simulink model "difflinrelay"  (Simulink 8.5)
settings: Solver=ode45  StartTime=0.0  StopTime=0.01  RelTol=1e-3
values from neighbouring files (symbols this model uses):
  n = abs(fix(dif/360))    [DE_12.m]
undefined symbols (not defined in the file or in its folder): b, den, dx, flagc, m, minx, num
libraries: elements x21, simulink_extras x9
(part 1 of 2)
settings Model: Creator=PC  LastModifiedBy=PC  ExtModeTrigMode=oneshot  ExtModeArmWhenConnect=off
settings DataIOCC: LimitDataPoints=off
settings OptimizationCC: BlockReduction=off  BooleanDataType=off  ExpressionDepthLimit=128
settings DebuggingCC: SaveWithParameterizedLinksMsg=none  SignalResolutionControl=TryResolveAllWithWarning  MultiTaskDSMMsg=warning  MultiTaskCondExecSysMsg=none  FcnCallInpInsideContextMsg=EnableAllAsError  StateNameClashWarn=none  StrictBusMsg=None
settings HardwareCC: TargetUnknown=on

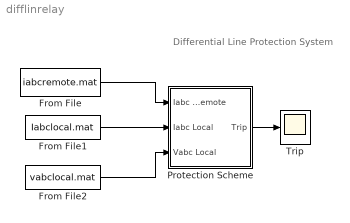
== system difflinrelay ==
  note: Differential Line Protection System
  From File : FromFile  FileName=iabcremote.mat  SampleTime=0
  From File1 : FromFile  FileName=Iabclocal.mat  SampleTime=0
  From File2 : FromFile  FileName=vabclocal.mat  SampleTime=0
  Protection Scheme : Subsystem  mask{bias=[ 0 0;1 0.5 ;3 0.8; 5 4; 7 4.2 ; 8 4.22], Cpg=1e-6, Cpp=1e-7, zone1=[0 0 ;1 0; 1 1; 0.5 1], zone2=[0 0; 2 0; 2 2; 0 2], zone3=[0 0; 3 0; 3 3 ;0 3], zone4=[0 0; 4 0; 5 4; 1 5], reversezone=[0 0; -1 0; -1 -1; 0 -1], delay=[0.001 0.002 0.003 0.001]}
      mask prompts: bias "Bias Characteristic"; Cpg "Capacitance between phase and ground (F)"; Cpp "Mutual Capacitance between phases (F)"; zone1 "Back-up protection zone 1:"; zone2 "Back-up protection zone 2"; zone3 "Back-up protection zone 3"; zone4 "Back-up protection zone 4"; reversezone "Back-up protection reverse zone"; delay "Delay times for zone protection [Z2 Z3 Z4 Reverse]"
  Trip : Scope
      settings: TickLabels=on  TimeRange=0.01  YMin=0  YMax=1.5
  wires:
  Protection Scheme/1(Trip) -> Trip/1
  From File2/1 -> Protection Scheme/3(Vabc Local)
  From File1/1 -> Protection Scheme/2(Iabc Local)
  From File/1 -> Protection Scheme/1(Iabc Remote)

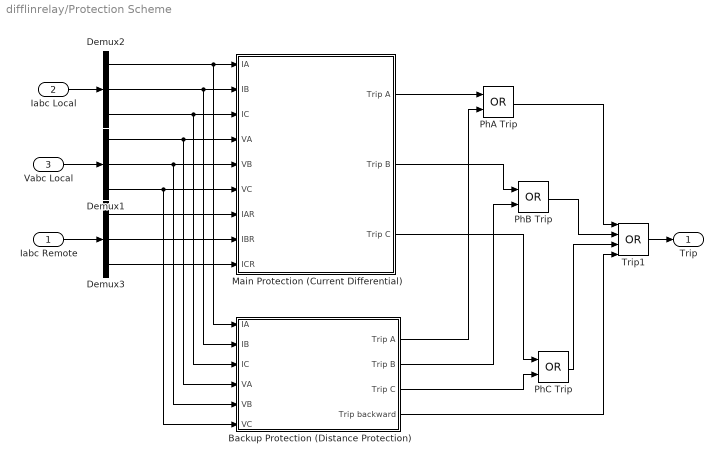
== system difflinrelay/Protection Scheme ==
  Iabc Remote : Inport
  Iabc Local : Inport  Port=2
  Vabc Local : Inport  Port=3
  Backup Protection (Distance Protection) : Subsystem
  Demux1 : Demux  Outputs=3
  Demux2 : Demux  Outputs=3
  Demux3 : Demux  Outputs=3
  Main Protection (Current Differential) : Subsystem
  PhA Trip : Logic  Operator=OR
  PhB Trip : Logic  Operator=OR
  PhC Trip : Logic  Operator=OR
  Trip1 : Logic  Operator=OR  Inputs=4
  Trip : Outport
  wires:
  Vabc Local/1 -> Demux1/1
  Iabc Local/1 -> Demux2/1
  Iabc Remote/1 -> Demux3/1
  Trip1/1 -> Trip/1
  PhA Trip/1 -> Trip1/1
  PhB Trip/1 -> Trip1/2
  PhC Trip/1 -> Trip1/3
  Backup Protection (Distance Protection)/1(Trip A) -> PhA Trip/2
  Backup Protection (Distance Protection)/2(Trip B) -> PhB Trip/2
  Backup Protection (Distance Protection)/3(Trip C) -> PhC Trip/2
  Main Protection (Current Differential)/1(Trip A) -> PhA Trip/1
  Main Protection (Current Differential)/2(Trip B) -> PhB Trip/1
  Main Protection (Current Differential)/3(Trip C) -> PhC Trip/1
  Demux3/1 -> Main Protection (Current Differential)/7(IAR)
  Demux3/2 -> Main Protection (Current Differential)/8(IBR)
  Demux3/3 -> Main Protection (Current Differential)/9(ICR)
  Demux2/1 -> Main Protection (Current Differential)/1(IA), Backup Protection (Distance Protection)/1(IA)
  Demux2/2 -> Main Protection (Current Differential)/2(IB), Backup Protection (Distance Protection)/2(IB)
  Demux2/3 -> Main Protection (Current Differential)/3(IC), Backup Protection (Distance Protection)/3(IC)
  Demux1/1 -> Main Protection (Current Differential)/4(VA), Backup Protection (Distance Protection)/4(VA)
  Demux1/2 -> Main Protection (Current Differential)/5(VB), Backup Protection (Distance Protection)/5(VB)
  Demux1/3 -> Main Protection (Current Differential)/6(VC), Backup Protection (Distance Protection)/6(VC)
  Backup Protection (Distance Protection)/4(Trip backward) -> Trip1/4

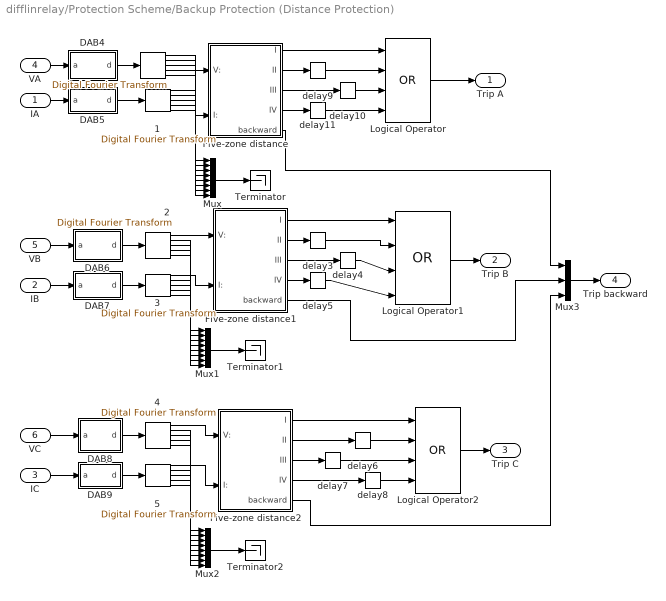
== system difflinrelay/Protection Scheme/Backup Protection (Distance Protection) ==
  IA : Inport
  IB : Inport  Port=2
  IC : Inport  Port=3
  VA : Inport  Port=4
  VB : Inport  Port=5
  VC : Inport  Port=6
   {,1..5} (6 alike) : elements/   fo=60  window_size=40  harmonic=[1 2 3 4 5]
  DAB4 : Subsystem  mask(Data Adquisition Board){filter=off, approx=Bessel, order=2, numerator=[], denominator=[], freq=180, resdis=off, vertres=12, xmax=10, winsize=40, G=1.0, fs=60*40}
      mask prompts: filter "Disable Analog Filter"; approx "Filter approximation"; numerator "Free expression filter: numerator(descending order of s)"; denominator "Free expression filter: denominator:"; freq "Cut-off frequency"; resdis "Disable Vertical Resolution"; vertres "Vertical Resolution: No. of bits"; xmax "Vertical Resolution: signal range"; winsize "Window size"; G "Gain"; fs "Sampling frequency"
      mask help: Performs analog filtering, signal conditioning and sampling. A single signal is the input, a buffer with the signal samples is the output. The options include analog filter enable/disable switch, type, order and cut-off frequency of the analog filter, conditioning gain, sampling frequency, number of bits, the length of the buffer.
      mask init:
      | dab1
      mask TypeOptions approx: Bessel | Tschebyscheff | Butterworth | free expression
      mask TypeOptions order: 2 | 3 | 4
      mask TypeOptions vertres: 8 | 12 | 16
      mask Display: disp('DAB')
  DAB5 : Subsystem  mask(Data Adquisition Board){filter=off, approx=Bessel, order=2, numerator=[], denominator=[], freq=180, resdis=off, vertres=12, xmax=10, winsize=40, G=1.0, fs=60*40}
      mask prompts: filter "Disable Analog Filter"; approx "Filter approximation"; numerator "Free expression filter: numerator(descending order of s)"; denominator "Free expression filter: denominator:"; freq "Cut-off frequency"; resdis "Disable Vertical Resolution"; vertres "Vertical Resolution: No. of bits"; xmax "Vertical Resolution: signal range"; winsize "Window size"; G "Gain"; fs "Sampling frequency"
      mask help: Performs analog filtering, signal conditioning and sampling. A single signal is the input, a buffer with the signal samples is the output. The options include analog filter enable/disable switch, type, order and cut-off frequency of the analog filter, conditioning gain, sampling frequency, number of bits, the length of the buffer.
      mask init:
      | dab1
      mask TypeOptions approx: Bessel | Tschebyscheff | Butterworth | free expression
      mask TypeOptions order: 2 | 3 | 4
      mask TypeOptions vertres: 8 | 12 | 16
      mask Display: disp('DAB')
  DAB6 : Subsystem  mask(Data Adquisition Board){filter=off, approx=Bessel, order=2, numerator=[], denominator=[], freq=180, resdis=off, vertres=12, xmax=10, winsize=40, G=1.0, fs=60*40}
      mask prompts: filter "Disable Analog Filter"; approx "Filter approximation"; numerator "Free expression filter: numerator(descending order of s)"; denominator "Free expression filter: denominator:"; freq "Cut-off frequency"; resdis "Disable Vertical Resolution"; vertres "Vertical Resolution: No. of bits"; xmax "Vertical Resolution: signal range"; winsize "Window size"; G "Gain"; fs "Sampling frequency"
      mask help: Performs analog filtering, signal conditioning and sampling. A single signal is the input, a buffer with the signal samples is the output. The options include analog filter enable/disable switch, type, order and cut-off frequency of the analog filter, conditioning gain, sampling frequency, number of bits, the length of the buffer.
      mask init:
      | dab1
      mask TypeOptions approx: Bessel | Tschebyscheff | Butterworth | free expression
      mask TypeOptions order: 2 | 3 | 4
      mask TypeOptions vertres: 8 | 12 | 16
      mask Display: disp('DAB')
  DAB7 : Subsystem  mask(Data Adquisition Board){filter=off, approx=Bessel, order=2, numerator=[], denominator=[], freq=180, resdis=off, vertres=12, xmax=10, winsize=40, G=1.0, fs=60*40}
      mask prompts: filter "Disable Analog Filter"; approx "Filter approximation"; numerator "Free expression filter: numerator(descending order of s)"; denominator "Free expression filter: denominator:"; freq "Cut-off frequency"; resdis "Disable Vertical Resolution"; vertres "Vertical Resolution: No. of bits"; xmax "Vertical Resolution: signal range"; winsize "Window size"; G "Gain"; fs "Sampling frequency"
      mask help: Performs analog filtering, signal conditioning and sampling. A single signal is the input, a buffer with the signal samples is the output. The options include analog filter enable/disable switch, type, order and cut-off frequency of the analog filter, conditioning gain, sampling frequency, number of bits, the length of the buffer.
      mask init:
      | dab1
      mask TypeOptions approx: Bessel | Tschebyscheff | Butterworth | free expression
      mask TypeOptions order: 2 | 3 | 4
      mask TypeOptions vertres: 8 | 12 | 16
      mask Display: disp('DAB')
  DAB8 : Subsystem  mask(Data Adquisition Board){filter=off, approx=Bessel, order=2, numerator=[], denominator=[], freq=180, resdis=off, vertres=12, xmax=10, winsize=40, G=1.0, fs=60*40}
      mask prompts: filter "Disable Analog Filter"; approx "Filter approximation"; numerator "Free expression filter: numerator(descending order of s)"; denominator "Free expression filter: denominator:"; freq "Cut-off frequency"; resdis "Disable Vertical Resolution"; vertres "Vertical Resolution: No. of bits"; xmax "Vertical Resolution: signal range"; winsize "Window size"; G "Gain"; fs "Sampling frequency"
      mask help: Performs analog filtering, signal conditioning and sampling. A single signal is the input, a buffer with the signal samples is the output. The options include analog filter enable/disable switch, type, order and cut-off frequency of the analog filter, conditioning gain, sampling frequency, number of bits, the length of the buffer.
      mask init:
      | dab1
      mask TypeOptions approx: Bessel | Tschebyscheff | Butterworth | free expression
      mask TypeOptions order: 2 | 3 | 4
      mask TypeOptions vertres: 8 | 12 | 16
      mask Display: disp('DAB')
  DAB9 : Subsystem  mask(Data Adquisition Board){filter=off, approx=Bessel, order=2, numerator=[], denominator=[], freq=180, resdis=off, vertres=12, xmax=10, winsize=40, G=1.0, fs=60*40}
      mask prompts: filter "Disable Analog Filter"; approx "Filter approximation"; numerator "Free expression filter: numerator(descending order of s)"; denominator "Free expression filter: denominator:"; freq "Cut-off frequency"; resdis "Disable Vertical Resolution"; vertres "Vertical Resolution: No. of bits"; xmax "Vertical Resolution: signal range"; winsize "Window size"; G "Gain"; fs "Sampling frequency"
      mask help: Performs analog filtering, signal conditioning and sampling. A single signal is the input, a buffer with the signal samples is the output. The options include analog filter enable/disable switch, type, order and cut-off frequency of the analog filter, conditioning gain, sampling frequency, number of bits, the length of the buffer.
      mask init:
      | dab1
      mask TypeOptions approx: Bessel | Tschebyscheff | Butterworth | free expression
      mask TypeOptions order: 2 | 3 | 4
      mask TypeOptions vertres: 8 | 12 | 16
      mask Display: disp('DAB')
  Five-zone distance : Subsystem
  Five-zone distance1 : Subsystem
  Five-zone distance2 : Subsystem
  Logical Operator : Logic  Operator=OR  Inputs=4
  Logical Operator1 : Logic  Operator=OR  Inputs=4
  Logical Operator2 : Logic  Operator=OR  Inputs=4
  Mux : Mux  Inputs=8
  Mux1 : Mux  Inputs=8
  Mux2 : Mux  Inputs=8
  Mux3 : Mux  Inputs=3
  Terminator : Terminator
  Terminator1 : Terminator
  Terminator2 : Terminator
  delay10 : TransportDelay  DelayTime=delay(2)
  delay11 : TransportDelay  DelayTime=delay(3)
  delay3 : TransportDelay  DelayTime=delay(1)
  delay4 : TransportDelay  DelayTime=delay(2)
  delay5 : TransportDelay  DelayTime=delay(3)
  delay6 : TransportDelay  DelayTime=delay(1)
  delay7 : TransportDelay  DelayTime=delay(2)
  delay8 : TransportDelay  DelayTime=delay(3)
  delay9 : TransportDelay  DelayTime=delay(1)
  Trip A : Outport
  Trip B : Outport  Port=2
  Trip C : Outport  Port=3
  Trip backward : Outport  Port=4
  wires:
  Five-zone distance1/1(I) -> Logical Operator1/1
  " 4"/1 -> Five-zone distance2/1(V:)
  DAB9/1(d) -> " 5"/1
  DAB8/1(d) -> " 4"/1
  VC/1 -> DAB8/1(a)
  IC/1 -> DAB9/1(a)
  Logical Operator2/1 -> Trip C/1
  " 2"/1 -> Five-zone distance1/1(V:)
  DAB7/1(d) -> " 3"/1
  DAB6/1(d) -> " 2"/1
  " 3"/1 -> Five-zone distance1/2(I:)
  Five-zone distance1/2(II) -> delay3/1
  Five-zone distance1/3(III) -> delay4/1
  Five-zone distance1/4(IV) -> delay5/1
  delay3/1 -> Logical Operator1/2
  delay4/1 -> Logical Operator1/3
  delay5/1 -> Logical Operator1/4
  VB/1 -> DAB6/1(a)
  IB/1 -> DAB7/1(a)
  Logical Operator1/1 -> Trip B/1
  " "/1 -> Five-zone distance/1(V:)
  DAB5/1(d) -> " 1"/1
  DAB4/1(d) -> " "/1
  " 1"/1 -> Five-zone distance/2(I:)
  Five-zone distance/1(I) -> Logical Operator/1
  VA/1 -> DAB4/1(a)
  IA/1 -> DAB5/1(a)
  Logical Operator/1 -> Trip A/1
  " "/3 -> Mux/1
  " "/2 -> Mux/2
  " "/4 -> Mux/3
  " "/5 -> Mux/4
  " 1"/2 -> Mux/5
  " 1"/3 -> Mux/6
  " 1"/4 -> Mux/7
  " 1"/5 -> Mux/8
  " 2"/2 -> Mux1/1
  " 2"/3 -> Mux1/2
  " 2"/4 -> Mux1/3
  " 2"/5 -> Mux1/4
  " 3"/2 -> Mux1/5
  " 3"/3 -> Mux1/6
  " 3"/4 -> Mux1/7
  " 3"/5 -> Mux1/8
  " 4"/3 -> Mux2/1
  " 4"/2 -> Mux2/2
  " 4"/4 -> Mux2/3
  " 4"/5 -> Mux2/4
  " 5"/2 -> Mux2/5
  " 5"/3 -> Mux2/6
  " 5"/4 -> Mux2/7
  " 5"/5 -> Mux2/8
  Five-zone distance/5(backward) -> Mux3/1
  Five-zone distance1/5(backward) -> Mux3/2
  " 5"/1 -> Five-zone distance2/2(I:)
  delay6/1 -> Logical Operator2/2
  delay7/1 -> Logical Operator2/3
  delay8/1 -> Logical Operator2/4
  Five-zone distance2/1(I) -> Logical Operator2/1
  Five-zone distance2/2(II) -> delay6/1
  Five-zone distance2/3(III) -> delay7/1
  Five-zone distance2/4(IV) -> delay8/1
  Five-zone distance2/5(backward) -> Mux3/3
  Five-zone distance/2(II) -> delay9/1
  delay9/1 -> Logical Operator/2
  Five-zone distance/3(III) -> delay10/1
  Five-zone distance/4(IV) -> delay11/1
  Mux/1 -> Terminator/1
  Mux1/1 -> Terminator1/1
  Mux2/1 -> Terminator2/1
  delay10/1 -> Logical Operator/3
  delay11/1 -> Logical Operator/4
  Mux3/1 -> Trip backward/1

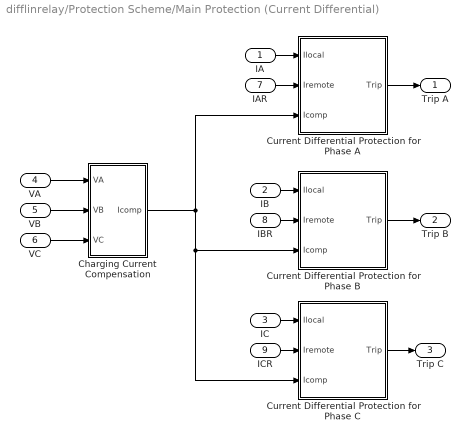
== system difflinrelay/Protection Scheme/Main Protection (Current Differential) ==
  IA : Inport
  IB : Inport  Port=2
  IC : Inport  Port=3
  VA : Inport  Port=4
  VB : Inport  Port=5
  VC : Inport  Port=6
  IAR : Inport  Port=7
  IBR : Inport  Port=8
  ICR : Inport  Port=9
  Charging Current Compensation : Subsystem
  Current Differential Protection for Phase A : Subsystem
  Current Differential Protection for Phase B : Subsystem
  Current Differential Protection for Phase C : Subsystem
  Trip A : Outport  InitialOutput=0
  Trip B : Outport  Port=2  InitialOutput=0
  Trip C : Outport  Port=3  InitialOutput=0
  wires:
  IA/1 -> Current Differential Protection for Phase A/1(Ilocal)
  IAR/1 -> Current Differential Protection for Phase A/2(Iremote)
  IB/1 -> Current Differential Protection for Phase B/1(Ilocal)
  Current Differential Protection for Phase C/1(Trip) -> Trip C/1
  Current Differential Protection for Phase A/1(Trip) -> Trip A/1
  Current Differential Protection for Phase B/1(Trip) -> Trip B/1
  VB/1 -> Charging Current Compensation/2(VB)
  IBR/1 -> Current Differential Protection for Phase B/2(Iremote)
  IC/1 -> Current Differential Protection for Phase C/1(Ilocal)
  VA/1 -> Charging Current Compensation/1(VA)
  VC/1 -> Charging Current Compensation/3(VC)
  ICR/1 -> Current Differential Protection for Phase C/2(Iremote)
  Charging Current Compensation/1(Icomp) -> Current Differential Protection for Phase A/3(Icomp), Current Differential Protection for Phase B/3(Icomp), Current Differential Protection for Phase C/3(Icomp)

== system difflinrelay/Protection Scheme/Backup Protection (Distance Protection)/DAB4 ==
  a : Inport
  AD & Buffer : S-Function  FunctionName=dab2  Parameters=winsize,fs,dx,resdis
  Analog Filter : TransferFcn  Numerator=num  Denominator=den
  Gain : Gain  Gain=G  SaturateOnIntegerOverflow=on  OutDataTypeStr=Inherit: Same as input  ParamDataTypeStr=Inherit: Same as input
  Zero-Order Hold : ZeroOrderHold  SampleTime=1/fs
  d : Outport  InitialOutput=[zeros(winsize,1)]
  wires:
  Analog Filter/1 -> Gain/1
  Gain/1 -> Zero-Order Hold/1
  Zero-Order Hold/1 -> AD & Buffer/1
  a/1 -> Analog Filter/1
  AD & Buffer/1 -> d/1

== system difflinrelay/Protection Scheme/Backup Protection (Distance Protection)/DAB5 ==
  a : Inport
  AD & Buffer : S-Function  FunctionName=dab2  Parameters=winsize,fs,dx,resdis
  Analog Filter : TransferFcn  Numerator=num  Denominator=den
  Gain : Gain  Gain=G  SaturateOnIntegerOverflow=on  OutDataTypeStr=Inherit: Same as input  ParamDataTypeStr=Inherit: Same as input
  Zero-Order Hold : ZeroOrderHold  SampleTime=1/fs
  d : Outport  InitialOutput=[zeros(winsize,1)]
  wires:
  AD & Buffer/1 -> d/1
  a/1 -> Analog Filter/1
  Zero-Order Hold/1 -> AD & Buffer/1
  Gain/1 -> Zero-Order Hold/1
  Analog Filter/1 -> Gain/1

== system difflinrelay/Protection Scheme/Backup Protection (Distance Protection)/DAB6 ==
  a : Inport
  AD & Buffer : S-Function  FunctionName=dab2  Parameters=winsize,fs,dx,resdis
  Analog Filter : TransferFcn  Numerator=num  Denominator=den
  Gain : Gain  Gain=G  SaturateOnIntegerOverflow=on  OutDataTypeStr=Inherit: Same as input  ParamDataTypeStr=Inherit: Same as input
  Zero-Order Hold : ZeroOrderHold  SampleTime=1/fs
  d : Outport  InitialOutput=[zeros(winsize,1)]
  wires:
  AD & Buffer/1 -> d/1
  a/1 -> Analog Filter/1
  Zero-Order Hold/1 -> AD & Buffer/1
  Gain/1 -> Zero-Order Hold/1
  Analog Filter/1 -> Gain/1

== system difflinrelay/Protection Scheme/Backup Protection (Distance Protection)/DAB7 ==
  a : Inport
  AD & Buffer : S-Function  FunctionName=dab2  Parameters=winsize,fs,dx,resdis
  Analog Filter : TransferFcn  Numerator=num  Denominator=den
  Gain : Gain  Gain=G  SaturateOnIntegerOverflow=on  OutDataTypeStr=Inherit: Same as input  ParamDataTypeStr=Inherit: Same as input
  Zero-Order Hold : ZeroOrderHold  SampleTime=1/fs
  d : Outport  InitialOutput=[zeros(winsize,1)]
  wires:
  Analog Filter/1 -> Gain/1
  Gain/1 -> Zero-Order Hold/1
  Zero-Order Hold/1 -> AD & Buffer/1
  a/1 -> Analog Filter/1
  AD & Buffer/1 -> d/1

== system difflinrelay/Protection Scheme/Backup Protection (Distance Protection)/DAB8 ==
  a : Inport
  AD & Buffer : S-Function  FunctionName=dab2  Parameters=winsize,fs,dx,resdis
  Analog Filter : TransferFcn  Numerator=num  Denominator=den
  Gain : Gain  Gain=G  SaturateOnIntegerOverflow=on  OutDataTypeStr=Inherit: Same as input  ParamDataTypeStr=Inherit: Same as input
  Zero-Order Hold : ZeroOrderHold  SampleTime=1/fs
  d : Outport  InitialOutput=[zeros(winsize,1)]
  wires:
  Analog Filter/1 -> Gain/1
  Gain/1 -> Zero-Order Hold/1
  Zero-Order Hold/1 -> AD & Buffer/1
  a/1 -> Analog Filter/1
  AD & Buffer/1 -> d/1

== system difflinrelay/Protection Scheme/Backup Protection (Distance Protection)/DAB9 ==
  a : Inport
  AD & Buffer : S-Function  FunctionName=dab2  Parameters=winsize,fs,dx,resdis
  Analog Filter : TransferFcn  Numerator=num  Denominator=den
  Gain : Gain  Gain=G  SaturateOnIntegerOverflow=on  OutDataTypeStr=Inherit: Same as input  ParamDataTypeStr=Inherit: Same as input
  Zero-Order Hold : ZeroOrderHold  SampleTime=1/fs
  d : Outport  InitialOutput=[zeros(winsize,1)]
  wires:
  AD & Buffer/1 -> d/1
  a/1 -> Analog Filter/1
  Zero-Order Hold/1 -> AD & Buffer/1
  Gain/1 -> Zero-Order Hold/1
  Analog Filter/1 -> Gain/1

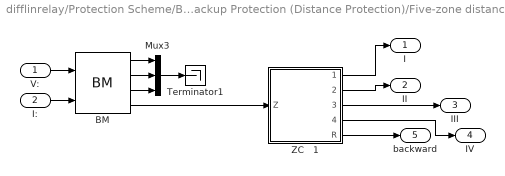
== system difflinrelay/Protection Scheme/Backup Protection (Distance Protection)/Five-zone distance ==
  V: : Inport
  I: : Inport  Port=2
  BM : elements/BM  tpostv=none  plenv=4  tposti=none  pleni=4  tposts=none  plens=4  tpostz=none  plenz=4
  Mux3 : Mux  Inputs=3
  Terminator1 : Terminator
  ZC   1 : Subsystem  mask(Zone Comparator){typez=Free expression, z1=zone1, z2=zone2, z3=zone3, z4=zone4, zr=reversezone, fs=4*60}
      mask prompts: typez "shape"; z1 "Zone 1"; z2 "Zone 2"; z3 "Zone 3"; z4 "Zone 4"; zr "Reverse Zone"; fs "Sampling frecuency (Hz):"
      mask help: This block performs the zone comparison. Its inputs are the resistance and reactance signals. Four forward and one backward zones are implemented. The output that corresponds to the zone where the impedance is located is set to one while the rest of the outputs are zero Either the mho or free expression characteristics may be set. For the mho characteristic, the zones are defined by specifying the center of each circle (all the circles are tangent to the origin). For the free expression, arrays with consecutive vertices specify the polygons for each zone.
      mask init:
      | zc1;
      mask TypeOptions typez: Mho characteristic | Free expression
      mask Display:
      | plot(x1(:,1),x1(:,2));
      | plot(x2(:,1),x2(:,2));
      | plot(x3(:,1),x3(:,2));
      | plot(x4(:,1),x4(:,2));
      | plot(xr(:,1),xr(:,2));
  I : Outport
  II : Outport  Port=2
  III : Outport  Port=3
  IV : Outport  Port=4
  backward : Outport  Port=5
  wires:
  I:/1 -> BM/2
  V:/1 -> BM/1
  BM/4 -> ZC   1/1(Z)
  BM/1 -> Mux3/1
  BM/2 -> Mux3/2
  BM/3 -> Mux3/3
  ZC   1/1(1) -> I/1
  ZC   1/2(2) -> II/1
  ZC   1/3(3) -> III/1
  ZC   1/4(4) -> IV/1
  ZC   1/5(R) -> backward/1
  Mux3/1 -> Terminator1/1

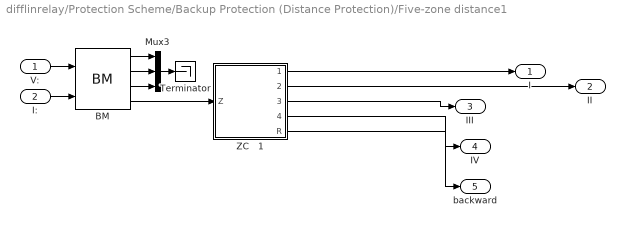
== system difflinrelay/Protection Scheme/Backup Protection (Distance Protection)/Five-zone distance1 ==
  V: : Inport
  I: : Inport  Port=2
  BM : elements/BM  tpostv=none  plenv=4  tposti=none  pleni=4  tposts=none  plens=4  tpostz=none  plenz=4
  Mux3 : Mux  Inputs=3
  Terminator : Terminator
  ZC   1 : Subsystem  mask(Zone Comparator){typez=Free expression, z1=zone1, z2=zone2, z3=zone3, z4=zone4, zr=reversezone, fs=4*60}
      mask prompts: typez "shape"; z1 "Zone 1"; z2 "Zone 2"; z3 "Zone 3"; z4 "Zone 4"; zr "Reverse Zone"; fs "Sampling frecuency (Hz):"
      mask help: This block performs the zone comparison. Its inputs are the resistance and reactance signals. Four forward and one backward zones are implemented. The output that corresponds to the zone where the impedance is located is set to one while the rest of the outputs are zero Either the mho or free expression characteristics may be set. For the mho characteristic, the zones are defined by specifying the center of each circle (all the circles are tangent to the origin). For the free expression, arrays with consecutive vertices specify the polygons for each zone.
      mask init:
      | zc1;
      mask TypeOptions typez: Mho characteristic | Free expression
      mask Display:
      | plot(x1(:,1),x1(:,2));
      | plot(x2(:,1),x2(:,2));
      | plot(x3(:,1),x3(:,2));
      | plot(x4(:,1),x4(:,2));
      | plot(xr(:,1),xr(:,2));
  I : Outport
  II : Outport  Port=2
  III : Outport  Port=3
  IV : Outport  Port=4
  backward : Outport  Port=5
  wires:
  ZC   1/5(R) -> backward/1
  ZC   1/4(4) -> IV/1
  ZC   1/3(3) -> III/1
  ZC   1/2(2) -> II/1
  ZC   1/1(1) -> I/1
  BM/3 -> Mux3/3
  BM/2 -> Mux3/2
  BM/1 -> Mux3/1
  BM/4 -> ZC   1/1(Z)
  V:/1 -> BM/1
  I:/1 -> BM/2
  Mux3/1 -> Terminator/1

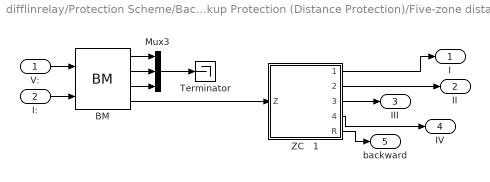
== system difflinrelay/Protection Scheme/Backup Protection (Distance Protection)/Five-zone distance2 ==
  V: : Inport
  I: : Inport  Port=2
  BM : elements/BM  tpostv=none  plenv=4  tposti=none  pleni=4  tposts=none  plens=4  tpostz=none  plenz=4
  Mux3 : Mux  Inputs=3
  Terminator : Terminator
  ZC   1 : Subsystem  mask(Zone Comparator){typez=Free expression, z1=zone1, z2=zone2, z3=zone3, z4=zone4, zr=reversezone, fs=4*60}
      mask prompts: typez "shape"; z1 "Zone 1"; z2 "Zone 2"; z3 "Zone 3"; z4 "Zone 4"; zr "Reverse Zone"; fs "Sampling frecuency (Hz):"
      mask help: This block performs the zone comparison. Its inputs are the resistance and reactance signals. Four forward and one backward zones are implemented. The output that corresponds to the zone where the impedance is located is set to one while the rest of the outputs are zero Either the mho or free expression characteristics may be set. For the mho characteristic, the zones are defined by specifying the center of each circle (all the circles are tangent to the origin). For the free expression, arrays with consecutive vertices specify the polygons for each zone.
      mask init:
      | zc1;
      mask TypeOptions typez: Mho characteristic | Free expression
      mask Display:
      | plot(x1(:,1),x1(:,2));
      | plot(x2(:,1),x2(:,2));
      | plot(x3(:,1),x3(:,2));
      | plot(x4(:,1),x4(:,2));
      | plot(xr(:,1),xr(:,2));
  I : Outport
  II : Outport  Port=2
  III : Outport  Port=3
  IV : Outport  Port=4
  backward : Outport  Port=5
  wires:
  I:/1 -> BM/2
  V:/1 -> BM/1
  BM/4 -> ZC   1/1(Z)
  BM/1 -> Mux3/1
  BM/2 -> Mux3/2
  BM/3 -> Mux3/3
  ZC   1/1(1) -> I/1
  ZC   1/2(2) -> II/1
  ZC   1/3(3) -> III/1
  ZC   1/4(4) -> IV/1
  ZC   1/5(R) -> backward/1
  Mux3/1 -> Terminator/1

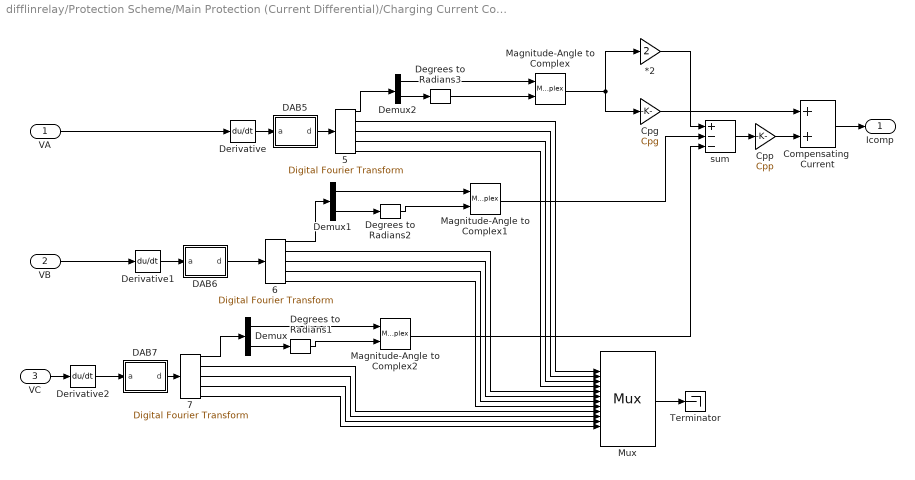
== system difflinrelay/Protection Scheme/Main Protection (Current Differential)/Charging Current Compensation ==
  VA : Inport
  VB : Inport  Port=2
  VC : Inport  Port=3
  " 5" : elements/   fo=60  window_size=40  harmonic=[1 2 3 4 5]
  " 6" : elements/   fo=60  window_size=40  harmonic=[1 2 3 4 5]
  " 7" : elements/   fo=60  window_size=40  harmonic=[1 2 3 4 5]
  *2 : Gain  Gain=2  SaturateOnIntegerOverflow=on  OutDataTypeStr=Inherit: Same as input  ParamDataTypeStr=Inherit: Same as input
  Compensating  Current : Sum  SaturateOnIntegerOverflow=on  InputSameDT=on  OutDataTypeStr=Inherit: Same as first input
  Cpg : Gain  Gain=Cpg  SaturateOnIntegerOverflow=on  OutDataTypeStr=Inherit: Same as input  ParamDataTypeStr=Inherit: Same as input
  Cpp : Gain  Gain=Cpp  SaturateOnIntegerOverflow=on  OutDataTypeStr=Inherit: Same as input  ParamDataTypeStr=Inherit: Same as input
  DAB5 : Subsystem  mask(Data Adquisition Board){filter=off, approx=Bessel, order=2, numerator=[], denominator=[], freq=180, resdis=off, vertres=12, xmax=10, winsize=40, G=1.0, fs=60*40}
      mask prompts: filter "Disable Analog Filter"; approx "Filter approximation"; numerator "Free expression filter: numerator(descending order of s)"; denominator "Free expression filter: denominator:"; freq "Cut-off frequency"; resdis "Disable Vertical Resolution"; vertres "Vertical Resolution: No. of bits"; xmax "Vertical Resolution: signal range"; winsize "Window size"; G "Gain"; fs "Sampling frequency"
      mask help: Performs analog filtering, signal conditioning and sampling. A single signal is the input, a buffer with the signal samples is the output. The options include analog filter enable/disable switch, type, order and cut-off frequency of the analog filter, conditioning gain, sampling frequency, number of bits, the length of the buffer.
      mask init:
      | dab1
      mask TypeOptions approx: Bessel | Tschebyscheff | Butterworth | free expression
      mask TypeOptions order: 2 | 3 | 4
      mask TypeOptions vertres: 8 | 12 | 16
      mask Display: disp('DAB')
  DAB6 : Subsystem  mask(Data Adquisition Board){filter=off, approx=Bessel, order=2, numerator=[], denominator=[], freq=180, resdis=off, vertres=12, xmax=10, winsize=40, G=1.0, fs=60*40}
      mask prompts: filter "Disable Analog Filter"; approx "Filter approximation"; numerator "Free expression filter: numerator(descending order of s)"; denominator "Free expression filter: denominator:"; freq "Cut-off frequency"; resdis "Disable Vertical Resolution"; vertres "Vertical Resolution: No. of bits"; xmax "Vertical Resolution: signal range"; winsize "Window size"; G "Gain"; fs "Sampling frequency"
      mask help: Performs analog filtering, signal conditioning and sampling. A single signal is the input, a buffer with the signal samples is the output. The options include analog filter enable/disable switch, type, order and cut-off frequency of the analog filter, conditioning gain, sampling frequency, number of bits, the length of the buffer.
      mask init:
      | dab1
      mask TypeOptions approx: Bessel | Tschebyscheff | Butterworth | free expression
      mask TypeOptions order: 2 | 3 | 4
      mask TypeOptions vertres: 8 | 12 | 16
      mask Display: disp('DAB')
  DAB7 : Subsystem  mask(Data Adquisition Board){filter=off, approx=Bessel, order=2, numerator=[], denominator=[], freq=180, resdis=off, vertres=12, xmax=10, winsize=40, G=1.0, fs=60*40}
      mask prompts: filter "Disable Analog Filter"; approx "Filter approximation"; numerator "Free expression filter: numerator(descending order of s)"; denominator "Free expression filter: denominator:"; freq "Cut-off frequency"; resdis "Disable Vertical Resolution"; vertres "Vertical Resolution: No. of bits"; xmax "Vertical Resolution: signal range"; winsize "Window size"; G "Gain"; fs "Sampling frequency"
      mask help: Performs analog filtering, signal conditioning and sampling. A single signal is the input, a buffer with the signal samples is the output. The options include analog filter enable/disable switch, type, order and cut-off frequency of the analog filter, conditioning gain, sampling frequency, number of bits, the length of the buffer.
      mask init:
      | dab1
      mask TypeOptions approx: Bessel | Tschebyscheff | Butterworth | free expression
      mask TypeOptions order: 2 | 3 | 4
      mask TypeOptions vertres: 8 | 12 | 16
      mask Display: disp('DAB')
  Degrees to Radians1 : simulink_extras/Transformations/Degrees to Radians
  Degrees to Radians2 : simulink_extras/Transformations/Degrees to Radians
  Degrees to Radians3 : simulink_extras/Transformations/Degrees to Radians
  Demux : Demux  Outputs=2
  Demux1 : Demux  Outputs=2
  Demux2 : Demux  Outputs=2
  Derivative : Derivative
  Derivative1 : Derivative
  Derivative2 : Derivative
  Magnitude-Angle to Complex : MagnitudeAngleToComplex
  Magnitude-Angle to Complex1 : MagnitudeAngleToComplex
  Magnitude-Angle to Complex2 : MagnitudeAngleToComplex
  Mux : Mux  Inputs=12
  Terminator : Terminator
  sum : Sum  Inputs=+--  SaturateOnIntegerOverflow=on  InputSameDT=on  OutDataTypeStr=Inherit: Same as first input
  Icomp : Outport
  wires:
  Degrees to Radians3/1 -> Magnitude-Angle to Complex/2
  Demux2/2 -> Degrees to Radians3/1
  Degrees to Radians2/1 -> Magnitude-Angle to Complex1/2
  Degrees to Radians1/1 -> Magnitude-Angle to Complex2/2
  Demux/2 -> Degrees to Radians1/1
  Magnitude-Angle to Complex2/1 -> sum/3
  Demux/1 -> Magnitude-Angle to Complex2/1
  Magnitude-Angle to Complex1/1 -> sum/2
  Magnitude-Angle to Complex/1 -> Cpg/1, *2/1
  Demux2/1 -> Magnitude-Angle to Complex/1
  " 6"/5 -> Mux/8
  " 6"/4 -> Mux/7
  " 6"/3 -> Mux/6
  " 6"/2 -> Mux/5
  " 7"/5 -> Mux/12
  " 7"/4 -> Mux/11
  " 7"/3 -> Mux/10
  " 7"/2 -> Mux/9
  VC/1 -> Derivative2/1
  DAB7/1(d) -> " 7"/1
  Derivative2/1 -> DAB7/1(a)
  Cpp/1 -> Compensating  Current/2
  *2/1 -> sum/1
  Compensating  Current/1 -> Icomp/1
  sum/1 -> Cpp/1
  " 5"/4 -> Mux/3
  " 5"/3 -> Mux/2
  " 5"/2 -> Mux/1
  VA/1 -> Derivative/1
  Cpg/1 -> Compensating  Current/1
  DAB5/1(d) -> " 5"/1
  Derivative/1 -> DAB5/1(a)
  " 5"/5 -> Mux/4
  Mux/1 -> Terminator/1
  VB/1 -> Derivative1/1
  " 6"/1 -> Demux1/1
  DAB6/1(d) -> " 6"/1
  Derivative1/1 -> DAB6/1(a)
  " 7"/1 -> Demux/1
  Demux1/1 -> Magnitude-Angle to Complex1/1
  Demux1/2 -> Degrees to Radians2/1
  " 5"/1 -> Demux2/1

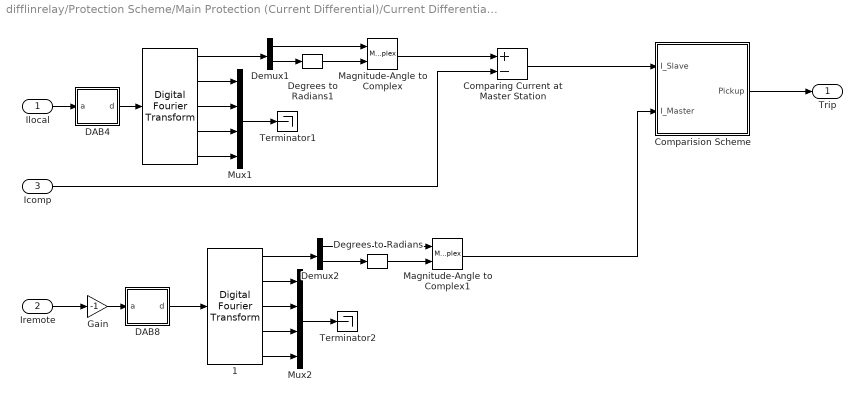
== system difflinrelay/Protection Scheme/Main Protection (Current Differential)/Current Differential Protection for Phase A ==
  Ilocal : Inport
  Iremote : Inport  Port=2
  Icomp : Inport  Port=3
  " " : elements/   fo=60  window_size=40  harmonic=[1 2 3 4 5]
  " 1" : elements/   fo=60  window_size=40  harmonic=[1 2 3 4 5]
  Comparing Current at Master Station : Sum  Inputs=+-  SaturateOnIntegerOverflow=on  InputSameDT=on  OutDataTypeStr=Inherit: Same as first input
  Comparision Scheme : Subsystem
  DAB4 : Subsystem  mask(Data Adquisition Board){filter=off, approx=Bessel, order=2, numerator=[], denominator=[], freq=180, resdis=off, vertres=12, xmax=10, winsize=40, G=1.0, fs=60*40}
      mask prompts: filter "Disable Analog Filter"; approx "Filter approximation"; numerator "Free expression filter: numerator(descending order of s)"; denominator "Free expression filter: denominator:"; freq "Cut-off frequency"; resdis "Disable Vertical Resolution"; vertres "Vertical Resolution: No. of bits"; xmax "Vertical Resolution: signal range"; winsize "Window size"; G "Gain"; fs "Sampling frequency"
      mask help: Performs analog filtering, signal conditioning and sampling. A single signal is the input, a buffer with the signal samples is the output. The options include analog filter enable/disable switch, type, order and cut-off frequency of the analog filter, conditioning gain, sampling frequency, number of bits, the length of the buffer.
      mask init:
      | dab1
      mask TypeOptions approx: Bessel | Tschebyscheff | Butterworth | free expression
      mask TypeOptions order: 2 | 3 | 4
      mask TypeOptions vertres: 8 | 12 | 16
      mask Display: disp('DAB')
  DAB8 : Subsystem  mask(Data Adquisition Board){filter=off, approx=Bessel, order=2, numerator=[], denominator=[], freq=180, resdis=off, vertres=12, xmax=10, winsize=40, G=1.0, fs=60*40}
      mask prompts: filter "Disable Analog Filter"; approx "Filter approximation"; numerator "Free expression filter: numerator(descending order of s)"; denominator "Free expression filter: denominator:"; freq "Cut-off frequency"; resdis "Disable Vertical Resolution"; vertres "Vertical Resolution: No. of bits"; xmax "Vertical Resolution: signal range"; winsize "Window size"; G "Gain"; fs "Sampling frequency"
      mask help: Performs analog filtering, signal conditioning and sampling. A single signal is the input, a buffer with the signal samples is the output. The options include analog filter enable/disable switch, type, order and cut-off frequency of the analog filter, conditioning gain, sampling frequency, number of bits, the length of the buffer.
      mask init:
      | dab1
      mask TypeOptions approx: Bessel | Tschebyscheff | Butterworth | free expression
      mask TypeOptions order: 2 | 3 | 4
      mask TypeOptions vertres: 8 | 12 | 16
      mask Display: disp('DAB')
  Degrees to Radians : simulink_extras/Transformations/Degrees to Radians
  Degrees to Radians1 : simulink_extras/Transformations/Degrees to Radians
  Demux1 : Demux  Outputs=2
  Demux2 : Demux  Outputs=2
  Gain : Gain  Gain=-1  SaturateOnIntegerOverflow=on  OutDataTypeStr=Inherit: Same as input  ParamDataTypeStr=Inherit: Same as input
  Magnitude-Angle to Complex : MagnitudeAngleToComplex
  Magnitude-Angle to Complex1 : MagnitudeAngleToComplex
  Mux1 : Mux
  Mux2 : Mux
  Terminator1 : Terminator
  Terminator2 : Terminator
  Trip : Outport  InitialOutput=0
  wires:
  Demux1/1 -> Magnitude-Angle to Complex/1
  " 1"/5 -> Mux2/4
  Comparing Current at Master Station/1 -> Comparision Scheme/1(I_Slave)
  Degrees to Radians1/1 -> Magnitude-Angle to Complex/2
  Demux1/2 -> Degrees to Radians1/1
  Icomp/1 -> Comparing Current at Master Station/2
  Magnitude-Angle to Complex/1 -> Comparing Current at Master Station/1
  Ilocal/1 -> DAB4/1(a)
  DAB4/1(d) -> " "/1
  Comparision Scheme/1(Pickup) -> Trip/1
  " "/1 -> Demux1/1
  Mux1/1 -> Terminator1/1
  " "/2 -> Mux1/1
  " "/3 -> Mux1/2
  " "/4 -> Mux1/3
  " "/5 -> Mux1/4
  Demux2/1 -> Magnitude-Angle to Complex1/1
  Degrees to Radians/1 -> Magnitude-Angle to Complex1/2
  Demux2/2 -> Degrees to Radians/1
  Magnitude-Angle to Complex1/1 -> Comparision Scheme/2(I_Master)
  DAB8/1(d) -> " 1"/1
  " 1"/1 -> Demux2/1
  Iremote/1 -> Gain/1
  Gain/1 -> DAB8/1(a)
  Mux2/1 -> Terminator2/1
  " 1"/3 -> Mux2/2
  " 1"/4 -> Mux2/3
  " 1"/2 -> Mux2/1

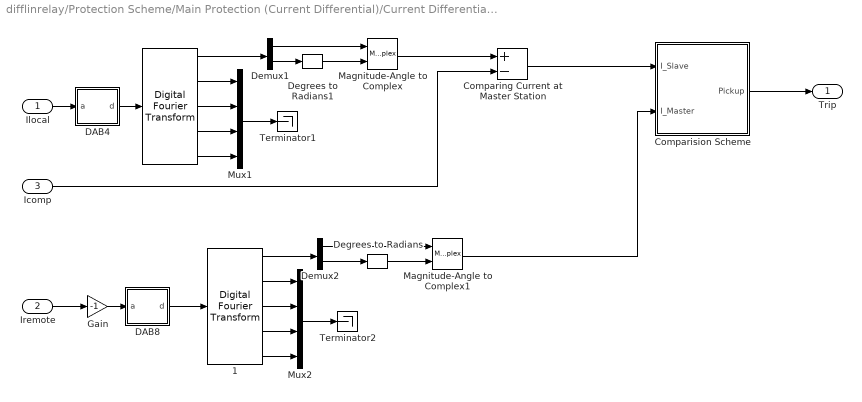
== system difflinrelay/Protection Scheme/Main Protection (Current Differential)/Current Differential Protection for Phase B ==
  Ilocal : Inport
  Iremote : Inport  Port=2
  Icomp : Inport  Port=3
  " " : elements/   fo=60  window_size=40  harmonic=[1 2 3 4 5]
  " 1" : elements/   fo=60  window_size=40  harmonic=[1 2 3 4 5]
  Comparing Current at Master Station : Sum  Inputs=+-  SaturateOnIntegerOverflow=on  InputSameDT=on  OutDataTypeStr=Inherit: Same as first input
  Comparision Scheme : Subsystem
  DAB4 : Subsystem  mask(Data Adquisition Board){filter=off, approx=Bessel, order=2, numerator=[], denominator=[], freq=180, resdis=off, vertres=12, xmax=10, winsize=40, G=1.0, fs=60*40}
      mask prompts: filter "Disable Analog Filter"; approx "Filter approximation"; numerator "Free expression filter: numerator(descending order of s)"; denominator "Free expression filter: denominator:"; freq "Cut-off frequency"; resdis "Disable Vertical Resolution"; vertres "Vertical Resolution: No. of bits"; xmax "Vertical Resolution: signal range"; winsize "Window size"; G "Gain"; fs "Sampling frequency"
      mask help: Performs analog filtering, signal conditioning and sampling. A single signal is the input, a buffer with the signal samples is the output. The options include analog filter enable/disable switch, type, order and cut-off frequency of the analog filter, conditioning gain, sampling frequency, number of bits, the length of the buffer.
      mask init:
      | dab1
      mask TypeOptions approx: Bessel | Tschebyscheff | Butterworth | free expression
      mask TypeOptions order: 2 | 3 | 4
      mask TypeOptions vertres: 8 | 12 | 16
      mask Display: disp('DAB')
  DAB8 : Subsystem  mask(Data Adquisition Board){filter=off, approx=Bessel, order=2, numerator=[], denominator=[], freq=180, resdis=off, vertres=12, xmax=10, winsize=40, G=1.0, fs=60*40}
      mask prompts: filter "Disable Analog Filter"; approx "Filter approximation"; numerator "Free expression filter: numerator(descending order of s)"; denominator "Free expression filter: denominator:"; freq "Cut-off frequency"; resdis "Disable Vertical Resolution"; vertres "Vertical Resolution: No. of bits"; xmax "Vertical Resolution: signal range"; winsize "Window size"; G "Gain"; fs "Sampling frequency"
      mask help: Performs analog filtering, signal conditioning and sampling. A single signal is the input, a buffer with the signal samples is the output. The options include analog filter enable/disable switch, type, order and cut-off frequency of the analog filter, conditioning gain, sampling frequency, number of bits, the length of the buffer.
      mask init:
      | dab1
      mask TypeOptions approx: Bessel | Tschebyscheff | Butterworth | free expression
      mask TypeOptions order: 2 | 3 | 4
      mask TypeOptions vertres: 8 | 12 | 16
      mask Display: disp('DAB')
  Degrees to Radians : simulink_extras/Transformations/Degrees to Radians
  Degrees to Radians1 : simulink_extras/Transformations/Degrees to Radians
  Demux1 : Demux  Outputs=2
  Demux2 : Demux  Outputs=2
  Gain : Gain  Gain=-1  SaturateOnIntegerOverflow=on  OutDataTypeStr=Inherit: Same as input  ParamDataTypeStr=Inherit: Same as input
  Magnitude-Angle to Complex : MagnitudeAngleToComplex
  Magnitude-Angle to Complex1 : MagnitudeAngleToComplex
  Mux1 : Mux
  Mux2 : Mux
  Terminator1 : Terminator
  Terminator2 : Terminator
  Trip : Outport  InitialOutput=0
  wires:
  " 1"/2 -> Mux2/1
  " 1"/4 -> Mux2/3
  " 1"/3 -> Mux2/2
  Mux2/1 -> Terminator2/1
  Gain/1 -> DAB8/1(a)
  Iremote/1 -> Gain/1
  " 1"/1 -> Demux2/1
  DAB8/1(d) -> " 1"/1
  Magnitude-Angle to Complex1/1 -> Comparision Scheme/2(I_Master)
  Demux2/2 -> Degrees to Radians/1
  Degrees to Radians/1 -> Magnitude-Angle to Complex1/2
  Demux2/1 -> Magnitude-Angle to Complex1/1
  " "/5 -> Mux1/4
  " "/4 -> Mux1/3
  " "/3 -> Mux1/2
  " "/2 -> Mux1/1
  Mux1/1 -> Terminator1/1
  " "/1 -> Demux1/1
  Comparision Scheme/1(Pickup) -> Trip/1
  DAB4/1(d) -> " "/1
  Ilocal/1 -> DAB4/1(a)
  Magnitude-Angle to Complex/1 -> Comparing Current at Master Station/1
  Icomp/1 -> Comparing Current at Master Station/2
  Demux1/2 -> Degrees to Radians1/1
  Degrees to Radians1/1 -> Magnitude-Angle to Complex/2
  Comparing Current at Master Station/1 -> Comparision Scheme/1(I_Slave)
  " 1"/5 -> Mux2/4
  Demux1/1 -> Magnitude-Angle to Complex/1

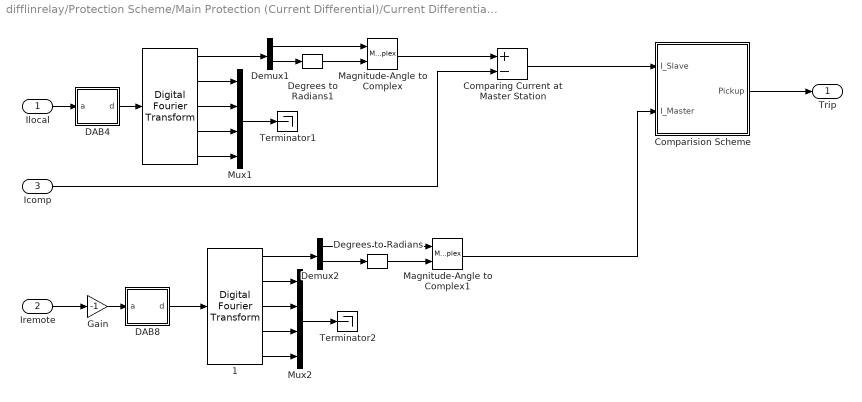
== system difflinrelay/Protection Scheme/Main Protection (Current Differential)/Current Differential Protection for Phase C ==
  Ilocal : Inport
  Iremote : Inport  Port=2
  Icomp : Inport  Port=3
  " " : elements/   fo=60  window_size=40  harmonic=[1 2 3 4 5]
  " 1" : elements/   fo=60  window_size=40  harmonic=[1 2 3 4 5]
  Comparing Current at Master Station : Sum  Inputs=+-  SaturateOnIntegerOverflow=on  InputSameDT=on  OutDataTypeStr=Inherit: Same as first input
  Comparision Scheme : Subsystem
  DAB4 : Subsystem  mask(Data Adquisition Board){filter=off, approx=Bessel, order=2, numerator=[], denominator=[], freq=180, resdis=off, vertres=12, xmax=10, winsize=40, G=1.0, fs=60*40}
      mask prompts: filter "Disable Analog Filter"; approx "Filter approximation"; numerator "Free expression filter: numerator(descending order of s)"; denominator "Free expression filter: denominator:"; freq "Cut-off frequency"; resdis "Disable Vertical Resolution"; vertres "Vertical Resolution: No. of bits"; xmax "Vertical Resolution: signal range"; winsize "Window size"; G "Gain"; fs "Sampling frequency"
      mask help: Performs analog filtering, signal conditioning and sampling. A single signal is the input, a buffer with the signal samples is the output. The options include analog filter enable/disable switch, type, order and cut-off frequency of the analog filter, conditioning gain, sampling frequency, number of bits, the length of the buffer.
      mask init:
      | dab1
      mask TypeOptions approx: Bessel | Tschebyscheff | Butterworth | free expression
      mask TypeOptions order: 2 | 3 | 4
      mask TypeOptions vertres: 8 | 12 | 16
      mask Display: disp('DAB')
  DAB8 : Subsystem  mask(Data Adquisition Board){filter=off, approx=Bessel, order=2, numerator=[], denominator=[], freq=180, resdis=off, vertres=12, xmax=10, winsize=40, G=1.0, fs=60*40}
      mask prompts: filter "Disable Analog Filter"; approx "Filter approximation"; numerator "Free expression filter: numerator(descending order of s)"; denominator "Free expression filter: denominator:"; freq "Cut-off frequency"; resdis "Disable Vertical Resolution"; vertres "Vertical Resolution: No. of bits"; xmax "Vertical Resolution: signal range"; winsize "Window size"; G "Gain"; fs "Sampling frequency"
      mask help: Performs analog filtering, signal conditioning and sampling. A single signal is the input, a buffer with the signal samples is the output. The options include analog filter enable/disable switch, type, order and cut-off frequency of the analog filter, conditioning gain, sampling frequency, number of bits, the length of the buffer.
      mask init:
      | dab1
      mask TypeOptions approx: Bessel | Tschebyscheff | Butterworth | free expression
      mask TypeOptions order: 2 | 3 | 4
      mask TypeOptions vertres: 8 | 12 | 16
      mask Display: disp('DAB')
  Degrees to Radians : simulink_extras/Transformations/Degrees to Radians
  Degrees to Radians1 : simulink_extras/Transformations/Degrees to Radians
  Demux1 : Demux  Outputs=2
  Demux2 : Demux  Outputs=2
  Gain : Gain  Gain=-1  SaturateOnIntegerOverflow=on  OutDataTypeStr=Inherit: Same as input  ParamDataTypeStr=Inherit: Same as input
  Magnitude-Angle to Complex : MagnitudeAngleToComplex
  Magnitude-Angle to Complex1 : MagnitudeAngleToComplex
  Mux1 : Mux
  Mux2 : Mux
  Terminator1 : Terminator
  Terminator2 : Terminator
  Trip : Outport  InitialOutput=0
  wires:
  Demux1/1 -> Magnitude-Angle to Complex/1
  " 1"/5 -> Mux2/4
  Comparing Current at Master Station/1 -> Comparision Scheme/1(I_Slave)
  Degrees to Radians1/1 -> Magnitude-Angle to Complex/2
  Demux1/2 -> Degrees to Radians1/1
  Icomp/1 -> Comparing Current at Master Station/2
  Magnitude-Angle to Complex/1 -> Comparing Current at Master Station/1
  Ilocal/1 -> DAB4/1(a)
  DAB4/1(d) -> " "/1
  Comparision Scheme/1(Pickup) -> Trip/1
  " "/1 -> Demux1/1
  Mux1/1 -> Terminator1/1
  " "/2 -> Mux1/1
  " "/3 -> Mux1/2
  " "/4 -> Mux1/3
  " "/5 -> Mux1/4
  Demux2/1 -> Magnitude-Angle to Complex1/1
  Degrees to Radians/1 -> Magnitude-Angle to Complex1/2
  Demux2/2 -> Degrees to Radians/1
  Magnitude-Angle to Complex1/1 -> Comparision Scheme/2(I_Master)
  DAB8/1(d) -> " 1"/1
  " 1"/1 -> Demux2/1
  Iremote/1 -> Gain/1
  Gain/1 -> DAB8/1(a)
  Mux2/1 -> Terminator2/1
  " 1"/3 -> Mux2/2
  " 1"/4 -> Mux2/3
  " 1"/2 -> Mux2/1

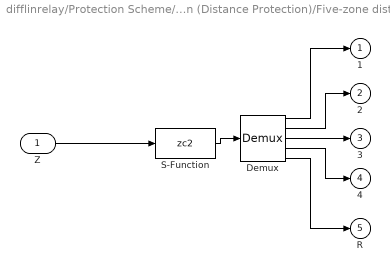
== system difflinrelay/Protection Scheme/Backup Protection (Distance Protection)/Five-zone distance/ZC   1 ==
  Z : Inport
  Demux : Demux  Outputs=5
  S-Function : S-Function  FunctionName=zc2  Parameters=z1,z2,z3,z4,zr,typez,fs,n,minx,flagc,m,b
  1 : Outport  InitialOutput=0
  2 : Outport  Port=2  InitialOutput=0
  3 : Outport  Port=3  InitialOutput=0
  4 : Outport  Port=4  InitialOutput=0
  R : Outport  Port=5  InitialOutput=0
  wires:
  S-Function/1 -> Demux/1
  Demux/1 -> 1/1
  Demux/2 -> 2/1
  Demux/3 -> 3/1
  Demux/4 -> 4/1
  Z/1 -> S-Function/1
  Demux/5 -> R/1

== system difflinrelay/Protection Scheme/Backup Protection (Distance Protection)/Five-zone distance1/ZC   1 ==
  Z : Inport
  Demux : Demux  Outputs=5
  S-Function : S-Function  FunctionName=zc2  Parameters=z1,z2,z3,z4,zr,typez,fs,n,minx,flagc,m,b
  1 : Outport  InitialOutput=0
  2 : Outport  Port=2  InitialOutput=0
  3 : Outport  Port=3  InitialOutput=0
  4 : Outport  Port=4  InitialOutput=0
  R : Outport  Port=5  InitialOutput=0
  wires:
  Demux/5 -> R/1
  Z/1 -> S-Function/1
  Demux/4 -> 4/1
  Demux/3 -> 3/1
  Demux/2 -> 2/1
  Demux/1 -> 1/1
  S-Function/1 -> Demux/1

== system difflinrelay/Protection Scheme/Backup Protection (Distance Protection)/Five-zone distance2/ZC   1 ==
  Z : Inport
  Demux : Demux  Outputs=5
  S-Function : S-Function  FunctionName=zc2  Parameters=z1,z2,z3,z4,zr,typez,fs,n,minx,flagc,m,b
  1 : Outport  InitialOutput=0
  2 : Outport  Port=2  InitialOutput=0
  3 : Outport  Port=3  InitialOutput=0
  4 : Outport  Port=4  InitialOutput=0
  R : Outport  Port=5  InitialOutput=0
  wires:
  S-Function/1 -> Demux/1
  Demux/1 -> 1/1
  Demux/2 -> 2/1
  Demux/3 -> 3/1
  Demux/4 -> 4/1
  Z/1 -> S-Function/1
  Demux/5 -> R/1

== system difflinrelay/Protection Scheme/Main Protection (Current Differential)/Charging Current Compensation/DAB5 ==
  a : Inport
  AD & Buffer : S-Function  FunctionName=dab2  Parameters=winsize,fs,dx,resdis
  Analog Filter : TransferFcn  Numerator=num  Denominator=den
  Gain : Gain  Gain=G  SaturateOnIntegerOverflow=on  OutDataTypeStr=Inherit: Same as input  ParamDataTypeStr=Inherit: Same as input
  Zero-Order Hold : ZeroOrderHold  SampleTime=1/fs
  d : Outport  InitialOutput=[zeros(winsize,1)]
  wires:
  Analog Filter/1 -> Gain/1
  Gain/1 -> Zero-Order Hold/1
  Zero-Order Hold/1 -> AD & Buffer/1
  a/1 -> Analog Filter/1
  AD & Buffer/1 -> d/1

== system difflinrelay/Protection Scheme/Main Protection (Current Differential)/Charging Current Compensation/DAB6 ==
  a : Inport
  AD & Buffer : S-Function  FunctionName=dab2  Parameters=winsize,fs,dx,resdis
  Analog Filter : TransferFcn  Numerator=num  Denominator=den
  Gain : Gain  Gain=G  SaturateOnIntegerOverflow=on  OutDataTypeStr=Inherit: Same as input  ParamDataTypeStr=Inherit: Same as input
  Zero-Order Hold : ZeroOrderHold  SampleTime=1/fs
  d : Outport  InitialOutput=[zeros(winsize,1)]
  wires:
  AD & Buffer/1 -> d/1
  a/1 -> Analog Filter/1
  Zero-Order Hold/1 -> AD & Buffer/1
  Gain/1 -> Zero-Order Hold/1
  Analog Filter/1 -> Gain/1

== system difflinrelay/Protection Scheme/Main Protection (Current Differential)/Charging Current Compensation/DAB7 ==
  a : Inport
  AD & Buffer : S-Function  FunctionName=dab2  Parameters=winsize,fs,dx,resdis
  Analog Filter : TransferFcn  Numerator=num  Denominator=den
  Gain : Gain  Gain=G  SaturateOnIntegerOverflow=on  OutDataTypeStr=Inherit: Same as input  ParamDataTypeStr=Inherit: Same as input
  Zero-Order Hold : ZeroOrderHold  SampleTime=1/fs
  d : Outport  InitialOutput=[zeros(winsize,1)]
  wires:
  Analog Filter/1 -> Gain/1
  Gain/1 -> Zero-Order Hold/1
  Zero-Order Hold/1 -> AD & Buffer/1
  a/1 -> Analog Filter/1
  AD & Buffer/1 -> d/1

== system difflinrelay/Protection Scheme/Main Protection (Current Differential)/Current Differential Protection for Phase A/Comparision Scheme ==
  I_Slave : Inport
  I_Master : Inport  Port=2
  Abs : Abs  SaturateOnIntegerOverflow=on
  Abs1 : Abs  SaturateOnIntegerOverflow=on
  Bias Characteristic1 : elements/Bias Characteristic  BC=bias  fs=60*20
  "Differential  Current " : Sum  SaturateOnIntegerOverflow=on  InputSameDT=on  OutDataTypeStr=Inherit: Same as first input
  Restraining  Current : Sum  Inputs=+-  SaturateOnIntegerOverflow=on  InputSameDT=on  OutDataTypeStr=Inherit: Same as first input
  Pickup : Outport
  wires:
  Restraining  Current/1 -> Abs1/1
  I_Slave/1 -> "Differential  Current "/1, Restraining  Current/1
  I_Master/1 -> "Differential  Current "/2, Restraining  Current/2
  Abs/1 -> Bias Characteristic1/1
  Bias Characteristic1/1 -> Pickup/1
  Abs1/1 -> Bias Characteristic1/2
  "Differential  Current "/1 -> Abs/1

== system difflinrelay/Protection Scheme/Main Protection (Current Differential)/Current Differential Protection for Phase A/DAB4 ==
  a : Inport
  AD & Buffer : S-Function  FunctionName=dab2  Parameters=winsize,fs,dx,resdis
  Analog Filter : TransferFcn  Numerator=num  Denominator=den
  Gain : Gain  Gain=G  SaturateOnIntegerOverflow=on  OutDataTypeStr=Inherit: Same as input  ParamDataTypeStr=Inherit: Same as input
  Zero-Order Hold : ZeroOrderHold  SampleTime=1/fs
  d : Outport  InitialOutput=[zeros(winsize,1)]
  wires:
  Analog Filter/1 -> Gain/1
  Gain/1 -> Zero-Order Hold/1
  Zero-Order Hold/1 -> AD & Buffer/1
  a/1 -> Analog Filter/1
  AD & Buffer/1 -> d/1
